simulink model "hw_torque_control_P_PI"  (R2021b)
settings: Solver=ode1  StartTime=0.0  StopTime=60  FixedStep=0.01  RelTol=1e-3  EnableMultiTasking=on
values from neighbouring files (symbols this model uses):
  D = (a*R*J - Kt^2)/R    (= -0.127706631544)    [motor_parameter.m]
  J = (Kt/(R*b))    (= 0.0439093113657)    [motor_parameter.m]
  kii = (J*(-Kt^2+kpo*R)*wn^2)/(Kt*(D^2+kpo^2+J^2*wn^2-2*J*kpo*wn*zeta+2*D*(kpo-J*wn*zeta)))    (= 4.59163436278)    [motor_parameter.m]
  kpi = -(D^2*R+J^2*R*wn^2+kpo*(Kt^2-2*J*R*wn*zeta)+D*(Kt^2+R*(kpo-2*J*wn*zeta))/(Kt*(D^2+kpo^2+J^2*wn^2-2*J*kpo*wn*zeta+2*D*(kpo-J*wn*zeta))))    (= 7.02770523889)    [motor_parameter.m]
  kpo = 10    [motor_parameter.m]
  Kt = 0.6777    [motor_parameter.m]
  R = 0.3826    [motor_parameter.m]
  Tc = (c*J)    (= 0.806614049787)    [motor_parameter.m]
libraries: arduinolib x6, arduinosensorlib x1
settings Model: ExtModeTrigDuration=2  Creator=ASUS  LastModifiedBy=ASUS
settings OptimizationCC: EnhancedBackFolding=on  PassReuseOutputArgsAs=Individual arguments  ZeroExternalMemoryAtStartup=off  ZeroInternalMemoryAtStartup=off  MaxStackSize=64  OptimizeBlockOrder=speed  DifferentSizesBufferReuse=on  OptimizationCustomize=off  EfficientTunableParamExpr=on
settings DebuggingCC: ParameterTunabilityLossMsg=error
settings HardwareCC: ProdBitPerInt=16  ProdBitPerPointer=16  ProdBitPerSizeT=16  ProdBitPerPtrDiffT=16  ProdLargestAtomicFloat=None  ProdWordSize=8  ProdHWDeviceType=Atmel->AVR
settings SFSimCC: MATLABDynamicMemAlloc=off
settings RTWCC: Description=Embedded Coder  SystemTargetFile=ert.tlc  HardwareBoard=Arduino Mega 2560  TemplateMakefile=ert_default_tmf  Toolchain=Arduino AVR  BuildConfiguration=Faster Runs
settings CodeAppCC: ForceParamTrailComments=on  IgnoreCustomStorageClasses=off  OperatorAnnotations=on  SimulinkDataObjDesc=on  SFDataObjDesc=on  InsertBlockDesc=on
settings ERTTargetCC: SupportContinuousTime=on  SupportVariableSizeSignals=on  ExtModeTransport=3  ExtModeStaticAlloc=on  ExtModeStaticAllocSize=2048  ExtModeMexFile=ext_xcp  ExtModeIntrfLevel=Level2 - Open

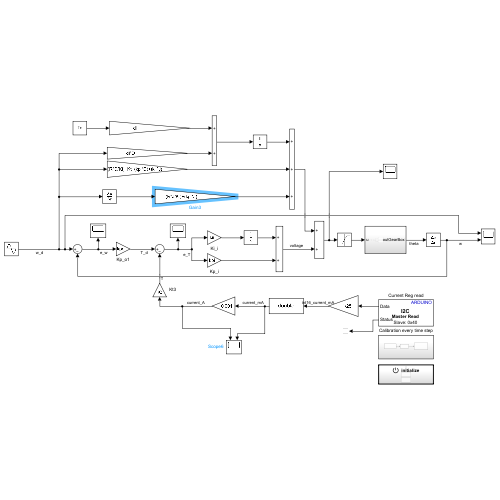
[thumbnail: Simulink's stored preview of the top-level diagram]
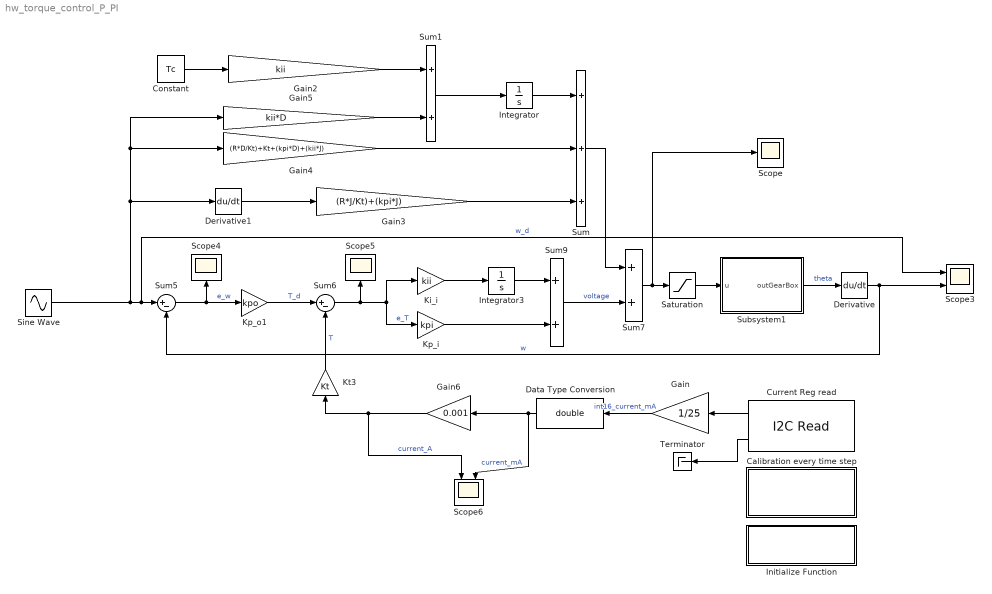
== system hw_torque_control_P_PI ==
  Calibration every time step : Subsystem  Priority=0
  Constant : Constant  Value=Tc
  Current Reg read : arduinolib/I2C Read  I2CModule=0  Mode=Master  SlaveAddress="hex2dec(\"0x40\")"  SlaveByteOrder=BigEndian  Direction=Receiver  RegisterAddressMode=on  RegisterAddress="hex2dec(\"0x04\")"  SlaveDataType=int16  DataLength=1  NoAck=off  RepeatedStart=off  OutputStatus=on  blockPlatform=ARDUINO  SampleTime=0.01
      settings: SourceProductBaseCode=ARDUINO
  Data Type Conversion : DataTypeConversion  OutDataTypeStr=double
  Derivative : Derivative
  Derivative1 : Derivative
  Gain : Gain  Gain=1/25
  Gain2 : Gain  Gain=kii
  Gain3 : Gain  Gain=(R*J/Kt)+(kpi*J)
  Gain4 : Gain  Gain=(R*D/Kt)+Kt+(kpi*D)+(kii*J)
  Gain5 : Gain  Gain=kii*D
  Gain6 : Gain  Gain=0.001
  Initialize Function : Subsystem  TreatAsAtomicUnit=on
  Integrator : Integrator
  Integrator3 : Integrator
  Ki_i : Gain  Gain=kii
  Kp_i : Gain  Gain=kpi
  Kp_o1 : Gain  Gain=kpo
  Kt3 : Gain  Gain=Kt
  Saturation : Saturate  UpperLimit=23  LowerLimit=-23
  Scope : Scope
  Scope3 : Scope  NumInputPorts=2
  Scope4 : Scope
  Scope5 : Scope
  Scope6 : Scope  NumInputPorts=2
  Sine Wave : Sin  Amplitude=5  Frequency=2*pi*0.4  SampleTime=0
  Subsystem1 : Subsystem
  Sum : Sum  Inputs=+++
  Sum1 : Sum
  Sum5 : Sum  Inputs=|+-
  Sum6 : Sum  Inputs=|+-
  Sum7 : Sum
  Sum9 : Sum
  Terminator : Terminator
  wires:
  Sum9/1 -> Sum7/2  "voltage"
  Sum5/1 -> Kp_o1/1, Scope4/1  "e_w"
  Sum6/1 -> Ki_i/1, Kp_i/1, Scope5/1  "e_T"
  Kp_i/1 -> Sum9/2
  Kp_o1/1 -> Sum6/1  "T_d"
  Ki_i/1 -> Integrator3/1
  Integrator3/1 -> Sum9/1
  Sum7/1 -> Scope/1, Saturation/1
  Sine Wave/1 -> Derivative1/1, Gain4/1, Gain5/1, Scope3/1, Sum5/1  "w_d"
  Constant/1 -> Gain2/1
  Gain2/1 -> Sum1/1
  Gain5/1 -> Sum1/2
  Sum1/1 -> Integrator/1
  Integrator/1 -> Sum/1
  Derivative1/1 -> Gain3/1
  Gain4/1 -> Sum/2
  Sum/1 -> Sum7/1
  Gain3/1 -> Sum/3
  Current Reg read/1 -> Gain/1
  Data Type Conversion/1 -> Gain6/1, Scope6/2  "current_mA"
  Gain/1 -> Data Type Conversion/1  "int16_current_mA"
  Current Reg read/2 -> Terminator/1
  Gain6/1 -> Scope6/1, Kt3/1  "current_A"
  Subsystem1/1(outGearBox) -> Derivative/1  "theta"
  Derivative/1 -> Scope3/2, Sum5/2  "w"
  Kt3/1 -> Sum6/2  "T"
  Saturation/1 -> Subsystem1/1(u)

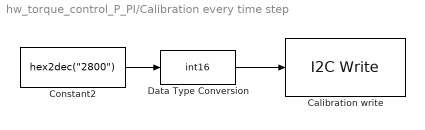
== system hw_torque_control_P_PI/Calibration every time step ==
  Calibration write : arduinolib/I2C Write  I2CModule=0  Mode=Master  SlaveAddress="uint8(hex2dec(\"0x40\"))"  SlaveByteOrder=BigEndian  Direction=Transmitter  RegisterAddressMode=on  RegisterAddress="uint8(hex2dec(\"0x05\"))"  SlaveDataType=uint8  DataLength=1  NoAck=off  RepeatedStart=off  OutputStatus=off  blockPlatform=ARDUINO
      settings: SourceProductBaseCode=ARDUINO
  Constant2 : Constant  Value="hex2dec(\"2800\")"
  Data Type Conversion : DataTypeConversion  OutDataTypeStr=int16
  wires:
  Constant2/1 -> Data Type Conversion/1
  Data Type Conversion/1 -> Calibration write/1

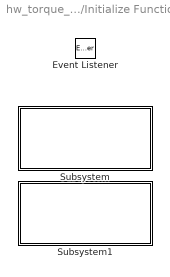
== system hw_torque_control_P_PI/Initialize Function ==
  Event Listener : EventListener  DisableCoverage=on  EventName=reset
  Subsystem : Subsystem  Priority=0
  Subsystem1 : Subsystem  Priority=1

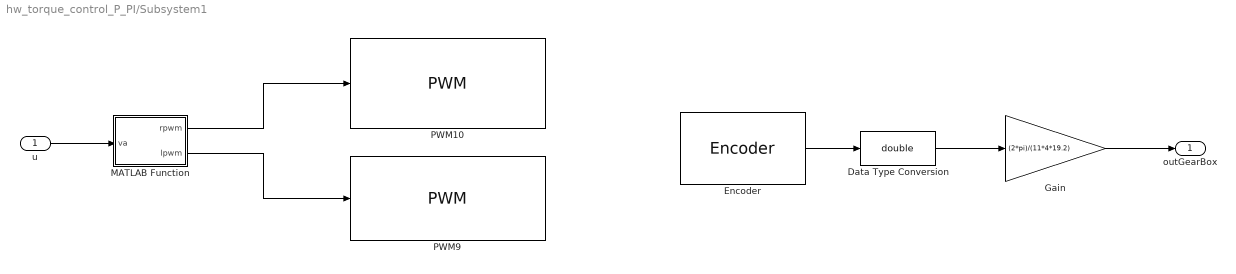
== system hw_torque_control_P_PI/Subsystem1 ==
  u : Inport
  Data Type Conversion : DataTypeConversion  OutDataTypeStr=double
  Encoder : arduinosensorlib/Encoder  InputA=2  InputB=3  Mode=No reset  SampleTime=-1
      settings: SourceProductBaseCode=ARDUINO
  Gain : Gain  Gain=(2*pi)/(11*4*19.2)
  MATLAB Function : MATLAB Function  TreatAsAtomicUnit=on
  PWM10 : arduinolib/PWM  pinNumber=8  frequencyType=Default  desiredFrequency=490.2  achievableFrequency=490.2
  PWM9 : arduinolib/PWM  pinNumber=9  frequencyType=Default  desiredFrequency=490.2  achievableFrequency=490.2
  outGearBox : Outport
  wires:
  Data Type Conversion/1 -> Gain/1
  Gain/1 -> outGearBox/1
  Encoder/1 -> Data Type Conversion/1
  u/1 -> MATLAB Function/1(va)
  MATLAB Function/1(rpwm) -> PWM10/1
  MATLAB Function/2(lpwm) -> PWM9/1

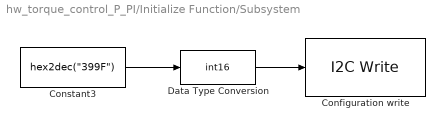
== system hw_torque_control_P_PI/Initialize Function/Subsystem ==
  Configuration write : arduinolib/I2C Write  I2CModule=0  Mode=Master  SlaveAddress="hex2dec(\"0x40\")"  SlaveByteOrder=BigEndian  Direction=Transmitter  RegisterAddressMode=on  RegisterAddress="hex2dec(\"0x00\")"  SlaveDataType=uint8  DataLength=1  NoAck=off  RepeatedStart=off  OutputStatus=off  blockPlatform=ARDUINO
      settings: SourceProductBaseCode=ARDUINO
  Constant3 : Constant  Value="hex2dec(\"399F\")"
  Data Type Conversion : DataTypeConversion  OutDataTypeStr=int16
  wires:
  Constant3/1 -> Data Type Conversion/1
  Data Type Conversion/1 -> Configuration write/1

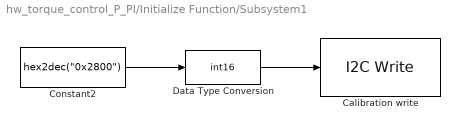
== system hw_torque_control_P_PI/Initialize Function/Subsystem1 ==
  Calibration write : arduinolib/I2C Write  I2CModule=0  Mode=Master  SlaveAddress="uint8(hex2dec(\"0x40\"))"  SlaveByteOrder=BigEndian  Direction=Transmitter  RegisterAddressMode=on  RegisterAddress="uint8(hex2dec(\"0x05\"))"  SlaveDataType=uint8  DataLength=1  NoAck=off  RepeatedStart=off  OutputStatus=off  blockPlatform=ARDUINO
      settings: SourceProductBaseCode=ARDUINO
  Constant2 : Constant  Value="hex2dec(\"0x2800\")"
  Data Type Conversion : DataTypeConversion  OutDataTypeStr=int16
  wires:
  Constant2/1 -> Data Type Conversion/1
  Data Type Conversion/1 -> Calibration write/1

== matlab function hw_torque_control_P_PI/Subsystem1/MATLAB Function ==
  data: va input; rpwm output; lpwm output
function [rpwm,lpwm] = fcn(va)

pwm = (va/24)*254;

if pwm > 0
    rpwm = pwm;
    lpwm = 0;
elseif pwm<0
    rpwm = 0;
    lpwm = abs(pwm);
else
    rpwm = 0;
    lpwm = 0;
end
